simulink model "prvi"  (R2017b)
settings: Solver=VariableStepAuto  StartTime=0.0  StopTime=10.0  RelTol=1e-3
values from neighbouring files (symbols this model uses):
  Ju = 0.0157    [podaci.m]
  K = (Uan-Ra*Ian)/(Nn*pi/30)    (= 0.908052161613)    [podaci.m]
  Ka = 1/Rau    (= 0.0585823081429)    [podaci.m]
  Ta = Lau/Rau    (= 0.0175981253661)    [podaci.m]
settings Model: Creator=USER  LastModifiedBy=USER

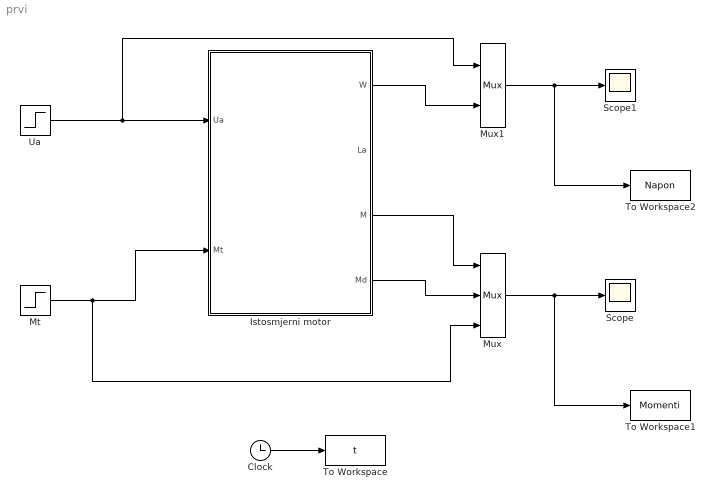
== system prvi ==
  Clock : Clock
  Istosmjerni motor : Subsystem
  Mt : Step  Time=5  Before=2  After=5  SampleTime=0
  Mux : Mux  Inputs=3
  Mux1 : Mux  Inputs=2
  Scope : Scope
  Scope1 : Scope
  To Workspace : ToWorkspace  VariableName=t  SampleTime=-1
  To Workspace1 : ToWorkspace  VariableName=Momenti  SampleTime=-1
  To Workspace2 : ToWorkspace  VariableName=Napon  SampleTime=-1
  Ua : Step  After=150  SampleTime=0
  wires:
  Ua/1 -> Mux1/1, Istosmjerni motor/1(Ua)
  Mt/1 -> Mux/3, Istosmjerni motor/2(Mt)
  Istosmjerni motor/4(Md) -> Mux/2
  Istosmjerni motor/3(M) -> Mux/1
  Mux/1 -> To Workspace1/1, Scope/1
  Istosmjerni motor/1(W) -> Mux1/2
  Mux1/1 -> To Workspace2/1, Scope1/1
  Clock/1 -> To Workspace/1

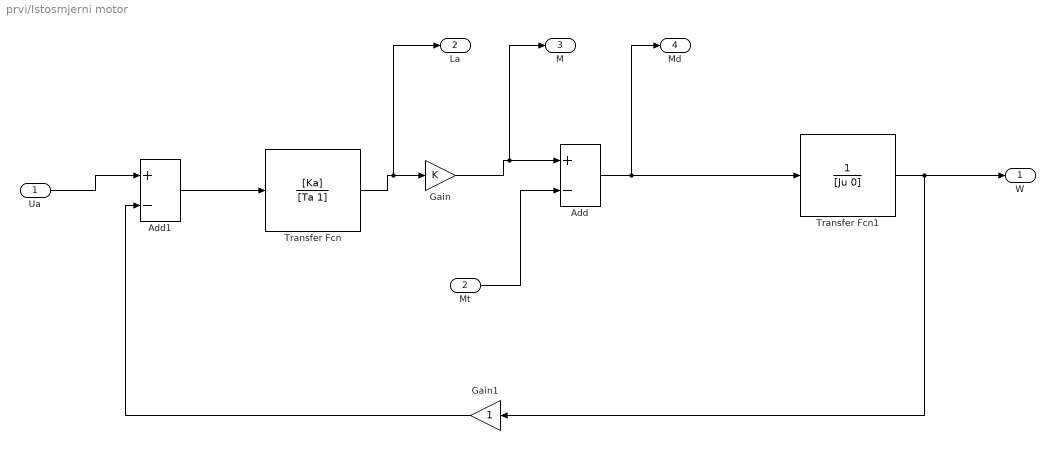
== system prvi/Istosmjerni motor ==
  Ua : Inport
  Mt : Inport  Port=2
  Add : Sum  Inputs=+-
  Add1 : Sum  Inputs=+-
  Gain : Gain  Gain=K
  Gain1 : Gain
  Transfer Fcn : TransferFcn  Numerator=[Ka]  Denominator=[Ta 1]
  Transfer Fcn1 : TransferFcn  Denominator=[Ju 0]
  W : Outport
  La : Outport  Port=2
  M : Outport  Port=3
  Md : Outport  Port=4
  wires:
  Add1/1 -> Transfer Fcn/1
  Gain1/1 -> Add1/2
  Transfer Fcn1/1 -> W/1, Gain1/1
  Transfer Fcn/1 -> La/1, Gain/1
  Ua/1 -> Add1/1
  Add/1 -> Md/1, Transfer Fcn1/1
  Gain/1 -> M/1, Add/1
  Mt/1 -> Add/2
